simulink model "PubIfCommonVIE_MDL_DS"  (R2020b)
settings: configuration reference "DspaceConfig" (kept outside this file)
PostLoadFcn:
  | if any(exist('dsrtsu_mdlpostloadfcn', 'file') ~= 0), dsrtsu_mdlpostloadfcn('Execute', bdroot); end
InitFcn:
  | , if any(exist('rtifpga_mdlclblib', 'file') ~= 0), rtifpga_mdlclblib('Init', bdroot); end,
  | , if any(exist('dsmpb_private', 'file') ~= 0), dsmpb_private('dsmpb_mdlclblib', 'Init', bdroot); end,
PreSaveFcn:
  | , if any(exist('dsmpb_private', 'file') ~= 0), dsmpb_private('dsmpb_mdlclblib', 'PreSave', bdroot); end,
CloseFcn:
  | , if any(exist('dsmpb_private', 'file') ~= 0), dsmpb_private('dsmpb_mdlclblib', 'Close', bdroot); end,
settings Model: RTICANMMDATA=struct('GeneralSetupData',struct('modelroot','C:\Users\GW00133806\Desktop\ADAS_Store\Project\V61_Autobox_Noa_Nofusion','generalsettings',struct('filesettings',struct('destfolder',struct('Name','RTICANMM_FILES','Check',1),'buildfolder',struct('Name','.','Check',1),'AbsDestfolder',struct('Name','C:\Users\GW00133806\Desktop\ADAS_Store\Project\V61_Autobox_Noa_Nofusion\RTICANMM_FILES'),'AbsBuildfolder',struct('Name','C:\Users\GW00133806\Desktop\ADAS_Store\Project\V61_Autobox_Noa_Nofusion'))),'options',struct('addpaths',1,'rmpaths',1,'addtrcexclusion',false,'cannavigator',struct('checkmonitoring',0),'show_usrtrc',0,'use_usrtrc',0),'advanced',struct('options',ones(1,100)),'MPSetup',{{}},'RTI',struct('Type','DSRT','Ver','4.4','Date','02-Nov-2020'),'modelname','PubIfCommonVIE_MDL_DS','block','PubIfCommonVIE_MDL_DS'))  DSRTSU_INTERNAL_RTIFPGA=170  Creator=GW00180895  LastModifiedBy=GW00133806
settings ConfigSetRef: SourceName=DspaceConfig  SourceLocation=Base Workspace

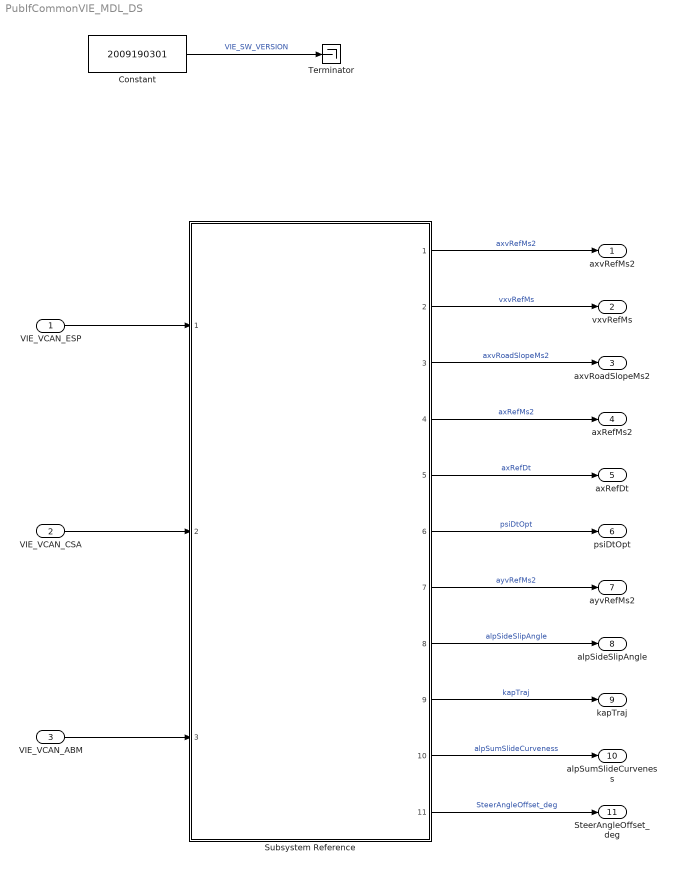
== system PubIfCommonVIE_MDL_DS ==
  VIE_VCAN_ESP : Inport  OutDataTypeStr=Bus: VCAN_ESP_MSG_BUS  PortDimensions=1  BusOutputAsStruct=on
  VIE_VCAN_CSA : Inport  Port=2  OutDataTypeStr=Bus: VCAN_CSA_MSG_BUS  PortDimensions=1  BusOutputAsStruct=on
  VIE_VCAN_ABM : Inport  Port=3  OutDataTypeStr=Bus: VCAN_ABM_MSG_BUS  PortDimensions=1  BusOutputAsStruct=on
  Constant : Constant  Value=2009190301  OutDataTypeStr=uint32
  Subsystem Reference : Subsystem  ReferencedSubsystem=PvtSubSys_VIE
  Terminator : Terminator
  axvRefMs2 : Outport  OutDataTypeStr=single  PortDimensions=1  BusOutputAsStruct=on
  vxvRefMs : Outport  Port=2  OutDataTypeStr=single  PortDimensions=1  BusOutputAsStruct=on
  axvRoadSlopeMs2 : Outport  Port=3  OutDataTypeStr=single  PortDimensions=1  BusOutputAsStruct=on
  axRefMs2 : Outport  Port=4  OutDataTypeStr=single  PortDimensions=1  BusOutputAsStruct=on
  axRefDt : Outport  Port=5  OutDataTypeStr=single  PortDimensions=1  BusOutputAsStruct=on
  psiDtOpt : Outport  Port=6  OutDataTypeStr=single  PortDimensions=1  BusOutputAsStruct=on
  ayvRefMs2 : Outport  Port=7  OutDataTypeStr=single  PortDimensions=1  BusOutputAsStruct=on
  alpSideSlipAngle : Outport  Port=8  OutDataTypeStr=single  PortDimensions=1  BusOutputAsStruct=on
  kapTraj : Outport  Port=9  OutDataTypeStr=single  PortDimensions=1  BusOutputAsStruct=on
  alpSumSlideCurveness : Outport  Port=10  OutDataTypeStr=single  PortDimensions=1  BusOutputAsStruct=on
  SteerAngleOffset_deg : Outport  Port=11  OutDataTypeStr=single  PortDimensions=1  BusOutputAsStruct=on
  wires:
  Subsystem Reference/3 -> axvRoadSlopeMs2/1  "axvRoadSlopeMs2"
  Subsystem Reference/2 -> vxvRefMs/1  "vxvRefMs"
  Subsystem Reference/4 -> axRefMs2/1  "axRefMs2"
  Subsystem Reference/1 -> axvRefMs2/1  "axvRefMs2"
  Subsystem Reference/5 -> axRefDt/1  "axRefDt"
  Subsystem Reference/6 -> psiDtOpt/1  "psiDtOpt"
  Subsystem Reference/7 -> ayvRefMs2/1  "ayvRefMs2"
  Subsystem Reference/8 -> alpSideSlipAngle/1  "alpSideSlipAngle"
  Subsystem Reference/9 -> kapTraj/1  "kapTraj"
  Subsystem Reference/10 -> alpSumSlideCurveness/1  "alpSumSlideCurveness"
  Subsystem Reference/11 -> SteerAngleOffset_deg/1  "SteerAngleOffset_deg"
  Constant/1 -> Terminator/1  "VIE_SW_VERSION"
  VIE_VCAN_CSA/1 -> Subsystem Reference/2
  VIE_VCAN_ABM/1 -> Subsystem Reference/3
  VIE_VCAN_ESP/1 -> Subsystem Reference/1
